simulink model "ctrl_systems_3"  (Simulink 10.2)
settings: Solver=ode45  StartTime=0.0  StopTime=365  MaxStep=0.01  RelTol=1e-3  EnableMultiTasking=on
values from neighbouring files (symbols this model uses):
  A = 10    [setup_Prac5.m]
  alpha = 0.1    [setup_Prac5.m]
  b1 = csvread('./DAE_ANN/ANN/Biases/30_04_21/lstm_ann_pi_standard_fix_noSo4_rnn_1__100_16_b_3.csv')    [init_PI_ann.m]    (also in init_PI_ann_hier.m = csvread('./DAE_ANN/ANN/Biases/12_05_21/lstm_ann_pi_standard_; init_PI_ann_hier_v2.m = csvread('./DAE_ANN/ANN/Biases/12_05_21/lstm_ann_pi_standard_; init_PI_ann_lab.m = csvread('./DAE_ANN/ANN/Biases/12_05_21/lstm_ann_pi_standard_)
  b2 = csvread('./DAE_ANN/ANN/Biases/30_04_21/lstm_ann_pi_standard_fix_noSo4_rnn_1__100_16_b_3.csv')    [init_PI_ann.m]    (also in init_PI_ann_hier.m = csvread('./DAE_ANN/ANN/Biases/12_05_21/lstm_ann_pi_standard_; init_PI_ann_hier_v2.m = csvread('./DAE_ANN/ANN/Biases/12_05_21/lstm_ann_pi_standard_; init_PI_ann_lab.m = csvread('./DAE_ANN/ANN/Biases/12_05_21/lstm_ann_pi_standard_)
  b_last = csvread('./DAE_ANN/ANN/Biases/12_05_21/lstm_ann_pi_standard_fix_noSo4_last__100_1_b_2.csv')'    [init_PI_ann_hier.m]    (also in init_PI_ann_hier_v2.m; init_PI_ann_lab.m)
  b_out = csvread('./DAE_ANN/ANN/Biases/30_04_21/lstm_ann_pi_standard_fix_noSo4_final__100_16_b_3.csv')    [init_PI_ann.m]    (also in init_PI_ann_hier.m = csvread('./DAE_ANN/ANN/Biases/12_05_21/lstm_ann_pi_standard_; init_PI_ann_hier_v2.m = csvread('./DAE_ANN/ANN/Biases/12_05_21/lstm_ann_pi_standard_; init_PI_ann_lab.m = csvread('./DAE_ANN/ANN/Biases/12_05_21/lstm_ann_pi_standard_)
  beta_ctrl = 0.3331    [setup_Prac5.m]
  k = k+1    (= 2)    [perf_risk.m]    (also in setup_Prac5.m = As*sqrt(2*g))
  K = 0.2294    [setup_Prac5.m]
  Kc_filter = 32.3841    [setup_Prac5.m]
  mean_scaler_dir = csvread('./DAE_ANN/ANN/Scalers/30_04_21_lstm_ann_pi_standard_fix_noSo4/mean_scaler_lstm_ann_pi_standard_fix_noSo4.csv')    [init_PI_ann.m]    (also in init_PI_ann_hier.m = csvread('./DAE_ANN/ANN/Scalers/12_05_21_lstm_ann_pi_standard; init_PI_ann_hier_v2.m = csvread('./DAE_ANN/ANN/Scalers/12_05_21_lstm_ann_pi_standard; setup_Prac5.m = [(Q/k)^2, 1.9756, 0.0000, 0]')
  mean_scaler_dir_out = csvread('./DAE_ANN/ANN/Scalers/30_04_21_lstm_ann_pi_standard_fix_noSo4/mean_scaler_lstm_ann_pi_standard_fix_noSo4_out.csv')    [init_PI_ann.m]    (also in init_PI_ann_hier.m = csvread('./DAE_ANN/ANN/Scalers/12_05_21_lstm_ann_pi_standard; init_PI_ann_hier_v2.m = csvread('./DAE_ANN/ANN/Scalers/12_05_21_lstm_ann_pi_standard; setup_Prac5.m = 0)
  n_layers = 1    [init_PI_ann.m]    (also in init_PI_ann_hier.m; init_PI_ann_hier_v2.m; init_PI_ann_lab.m)
  n_sw = 16    [init_PI_ann.m]    (also in init_PI_ann_hier.m = 1; init_PI_ann_hier_v2.m = 1; init_PI_ann_lab.m = 1)
  Q = 2    [setup_Prac5.m]
  So_mean = 2    [run_bsm1_PIANN_variable.m]    (also in setup_Prac5.m = 0.2)
  std_scaler_dir = csvread('./DAE_ANN/ANN/Scalers/30_04_21_lstm_ann_pi_standard_fix_noSo4/std_scaler_lstm_ann_pi_standard_fix_noSo4.csv')    [init_PI_ann.m]    (also in init_PI_ann_hier.m = csvread('./DAE_ANN/ANN/Scalers/12_05_21_lstm_ann_pi_standard; init_PI_ann_hier_v2.m = csvread('./DAE_ANN/ANN/Scalers/12_05_21_lstm_ann_pi_standard; setup_Prac5.m = [1, 0.7579, 0.05, 1]')
  std_scaler_dir_out = csvread('./DAE_ANN/ANN/Scalers/30_04_21_lstm_ann_pi_standard_fix_noSo4/std_scaler_lstm_ann_pi_standard_fix_noSo4_out.csv')    [init_PI_ann.m]    (also in init_PI_ann_hier.m = csvread('./DAE_ANN/ANN/Scalers/12_05_21_lstm_ann_pi_standard; init_PI_ann_hier_v2.m = csvread('./DAE_ANN/ANN/Scalers/12_05_21_lstm_ann_pi_standard; setup_Prac5.m = 1)
  T = 6.5201    [setup_Prac5.m]
  t_init = 7e-3    (= 0.007)    [run_bsm1.m]    (also in run_bsm1_PIANN_variable.m = 0.05)
  t_simulink = 1/96    (= 0.0104166666667)    [run_bsm1.m]    (also in run_bsm1_PIANN.m = -1; run_bsm1_PIANN_variable.m = 0; setup_Prac5.m = 0)
  Td_filter = 0.2776    [setup_Prac5.m]
  Ti_filter = 1.0264    [setup_Prac5.m]
  u1 = csvread('./DAE_ANN/ANN/Weights/30_04_21/lstm_ann_pi_standard_fix_noSo4_rnn_1__100_16_U_3.csv')    [init_PI_ann.m]    (also in init_PI_ann_hier.m = csvread('./DAE_ANN/ANN/Weights/12_05_21/lstm_ann_pi_standard; init_PI_ann_hier_v2.m = csvread('./DAE_ANN/ANN/Weights/12_05_21/lstm_ann_pi_standard)
  u2 = csvread('./DAE_ANN/ANN/Weights/30_04_21/lstm_ann_pi_standard_fix_noSo4_rnn_1__100_16_U_3.csv')    [init_PI_ann.m]    (also in init_PI_ann_hier.m = csvread('./DAE_ANN/ANN/Weights/12_05_21/lstm_ann_pi_standard; init_PI_ann_hier_v2.m = csvread('./DAE_ANN/ANN/Weights/12_05_21/lstm_ann_pi_standard)
  w1 = csvread('./DAE_ANN/ANN/Weights/30_04_21/lstm_ann_pi_standard_fix_noSo4_rnn_1__100_16_W_3.csv')    [init_PI_ann.m]    (also in init_PI_ann_hier.m = csvread('./DAE_ANN/ANN/Weights/12_05_21/lstm_ann_pi_standard; init_PI_ann_hier_v2.m = csvread('./DAE_ANN/ANN/Weights/12_05_21/lstm_ann_pi_standard; init_PI_ann_lab.m = csvread('./DAE_ANN/ANN/Weights/12_05_21/lstm_ann_pi_standard)
  w2 = csvread('./DAE_ANN/ANN/Weights/30_04_21/lstm_ann_pi_standard_fix_noSo4_rnn_1__100_16_W_3.csv')    [init_PI_ann.m]    (also in init_PI_ann_hier.m = csvread('./DAE_ANN/ANN/Weights/12_05_21/lstm_ann_pi_standard; init_PI_ann_hier_v2.m = csvread('./DAE_ANN/ANN/Weights/12_05_21/lstm_ann_pi_standard; init_PI_ann_lab.m = csvread('./DAE_ANN/ANN/Weights/12_05_21/lstm_ann_pi_standard)
  w_last = csvread('./DAE_ANN/ANN/Weights/12_05_21/lstm_ann_pi_standard_fix_noSo4_last__100_1_W_2.csv')    [init_PI_ann_hier.m]    (also in init_PI_ann_hier_v2.m; init_PI_ann_lab.m)
  w_out = csvread('./DAE_ANN/ANN/Weights/30_04_21/lstm_ann_pi_standard_fix_noSo4_final__100_16_W_3.csv')    [init_PI_ann.m]    (also in init_PI_ann_hier.m = csvread('./DAE_ANN/ANN/Weights/12_05_21/lstm_ann_pi_standard; init_PI_ann_hier_v2.m = csvread('./DAE_ANN/ANN/Weights/12_05_21/lstm_ann_pi_standard; init_PI_ann_lab.m = csvread('./DAE_ANN/ANN/Weights/12_05_21/lstm_ann_pi_standard)
  x0_ini = [2*(Q/k)^2  (Q/k)^2]    [setup_Prac5.m]
undefined symbols (not defined in the file or in its folder): Kc_zn, magnitude, Td_zn, Ti_zn
settings Model: Creator=carles  LastModifiedBy=win04
settings DataIOCC: OutputTimes=1
settings OptimizationCC: ExpressionDepthLimit=2147483647
settings DebuggingCC: SolverPrmCheckMsg=warning  StateNameClashWarn=warning
settings ConfigComp: CovSFcnEnable=off

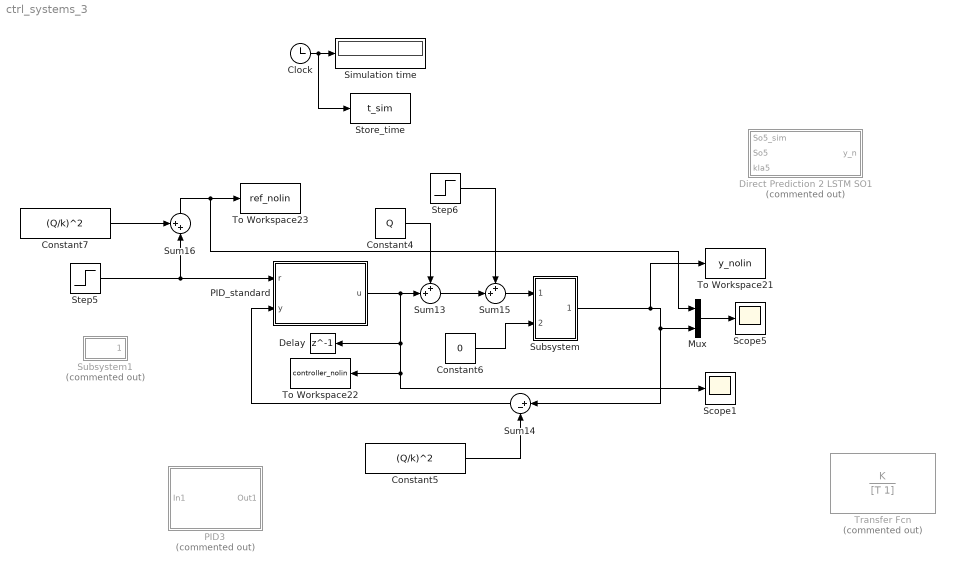
== system ctrl_systems_3 ==
  Clock : Clock
  Constant4 : Constant  Value=Q
  Constant5 : Constant  Value=(Q/k)^2
  Constant6 : Constant  Value=0
  Constant7 : Constant  Value=(Q/k)^2
  Delay : Delay  DelayLength=1  InitialCondition=0  SampleTime=0.0001
  Direct Prediction 2 LSTM SO1 : Subsystem  Commented=on
  Mux : Mux  Inputs=2
  PID3 : Subsystem  Commented=on
  PID_standard : Subsystem
  Scope1 : Scope
  Scope5 : Scope
  Simulation time : Display
  Step5 : Step  Time=5  After=0.2  SampleTime=0
  Step6 : Step  Time=30  After=0  SampleTime=0
  Store_time : ToWorkspace  VariableName=t_sim
  Subsystem : Subsystem
  Subsystem1 : Subsystem  Commented=on
  Sum13 : Sum  Inputs=++|
  Sum14 : Sum  Inputs=|+-
  Sum15 : Sum  Inputs=++|
  Sum16 : Sum  Inputs=++|
  To Workspace21 : ToWorkspace  VariableName=y_nolin  SampleTime=-1
  To Workspace22 : ToWorkspace  VariableName=controller_nolin  SampleTime=-1
  To Workspace23 : ToWorkspace  VariableName=ref_nolin  SampleTime=-1
  Transfer Fcn : TransferFcn  Commented=on  Numerator=K  Denominator=[T 1]
  wires:
  Subsystem/1(Out2) -> Sum14/1, Mux/2, To Workspace21/1
  Constant4/1 -> Sum13/1
  Constant5/1 -> Sum14/2
  PID_standard/1(u) -> Scope1/1, To Workspace22/1, Delay/1, Sum13/2
  Sum15/1 -> Subsystem/1(In1)
  Sum13/1 -> Sum15/2
  Step5/1 -> PID_standard/1(r), Sum16/2
  Step6/1 -> Sum15/1
  Sum16/1 -> Mux/1, To Workspace23/1
  Constant7/1 -> Sum16/1
  Clock/1 -> Store_time/1, Simulation time/1
  Sum14/1 -> PID_standard/2(y)
  Mux/1 -> Scope5/1
  Constant6/1 -> Subsystem/2(In2)

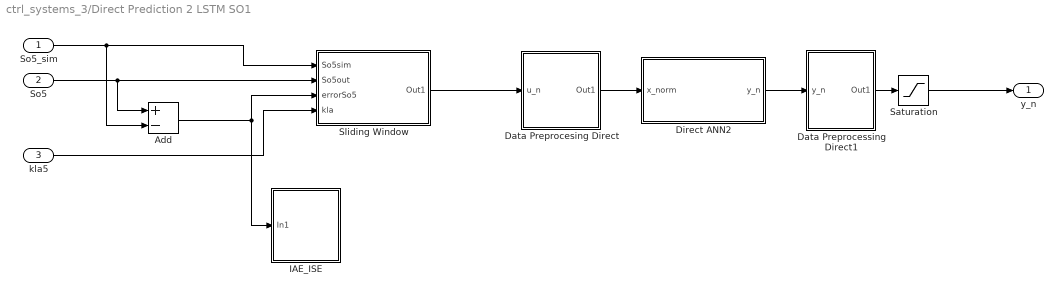
== system ctrl_systems_3/Direct Prediction 2 LSTM SO1 ==
  So5_sim : Inport
  So5 : Inport  Port=2
  kla5 : Inport  Port=3
  Add : Sum  Inputs=+-
  Data Preprocesing Direct : Subsystem
  Data Preprocessing Direct1 : Subsystem
  Direct ANN2 : Subsystem
  IAE_ISE : Subsystem
  Saturation : Saturate  UpperLimit=360  LowerLimit=-Q
  Sliding Window : Subsystem
  y_n : Outport  VectorParamsAs1DForOutWhenUnconnected=off
  wires:
  kla5/1 -> Sliding Window/4(kla)
  Add/1 -> Sliding Window/3(errorSo5), IAE_ISE/1(In1)
  So5/1 -> Sliding Window/2(So5out), Add/1
  So5_sim/1 -> Sliding Window/1(So5sim), Add/2
  Saturation/1 -> y_n/1
  Sliding Window/1(Out1) -> Data Preprocesing Direct/1(u_n)
  Data Preprocessing Direct1/1(Out1) -> Saturation/1
  Direct ANN2/1(y_n) -> Data Preprocessing Direct1/1(y_n)
  Data Preprocesing Direct/1(Out1) -> Direct ANN2/1(x_norm)

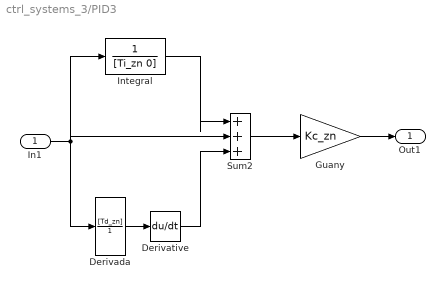
== system ctrl_systems_3/PID3 ==
  In1 : Inport
  Derivada : TransferFcn  Numerator=[Td_zn]  Denominator=[1]
  Derivative : Derivative
  Guany : Gain  Gain=Kc_zn
  Integral : TransferFcn  Denominator=[Ti_zn 0]
  Sum2 : Sum  Inputs=|+++
  Out1 : Outport
  wires:
  Derivative/1 -> Sum2/3
  Derivada/1 -> Derivative/1
  In1/1 -> Integral/1, Derivada/1, Sum2/2
  Integral/1 -> Sum2/1
  Sum2/1 -> Guany/1
  Guany/1 -> Out1/1

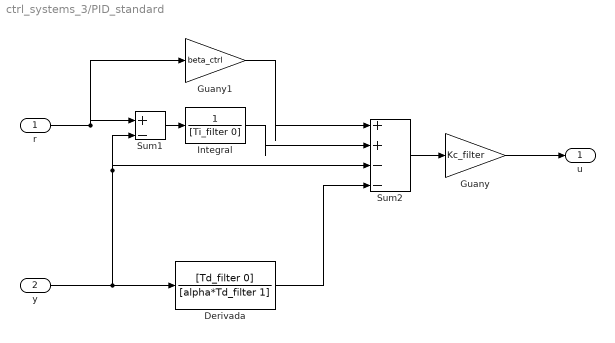
== system ctrl_systems_3/PID_standard ==
  r : Inport
  y : Inport  Port=2
  Derivada : TransferFcn  Numerator=[Td_filter 0]  Denominator=[alpha*Td_filter 1]
  Guany : Gain  Gain=Kc_filter
  Guany1 : Gain  Gain=beta_ctrl
  Integral : TransferFcn  Denominator=[Ti_filter 0]
  Sum1 : Sum  Inputs=|+-
  Sum2 : Sum  Inputs=|++--
  u : Outport
  wires:
  Guany/1 -> u/1
  Sum2/1 -> Guany/1
  r/1 -> Sum1/1, Guany1/1
  Guany1/1 -> Sum2/1
  Integral/1 -> Sum2/2
  y/1 -> Derivada/1, Sum2/3, Sum1/2
  Derivada/1 -> Sum2/4
  Sum1/1 -> Integral/1

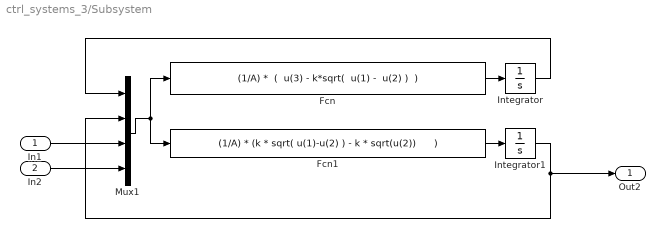
== system ctrl_systems_3/Subsystem ==
  In1 : Inport
  In2 : Inport  Port=2
  Fcn : Fcn  Expr="(1/A) *  (  u(3) - k*sqrt(  u(1) -  u(2) )  )"
  Fcn1 : Fcn  Expr="(1/A) * (k * sqrt( u(1)-u(2) ) - k * sqrt(u(2))      )"
  Integrator : Integrator  InitialCondition=x0_ini(1)
  Integrator1 : Integrator  InitialCondition=x0_ini(2)
  Mux1 : Mux
  Out2 : Outport
  wires:
  In1/1 -> Mux1/3
  In2/1 -> Mux1/4
  Integrator1/1 -> Out2/1, Mux1/2
  Integrator/1 -> Mux1/1
  Mux1/1 -> Fcn/1, Fcn1/1
  Fcn1/1 -> Integrator1/1
  Fcn/1 -> Integrator/1

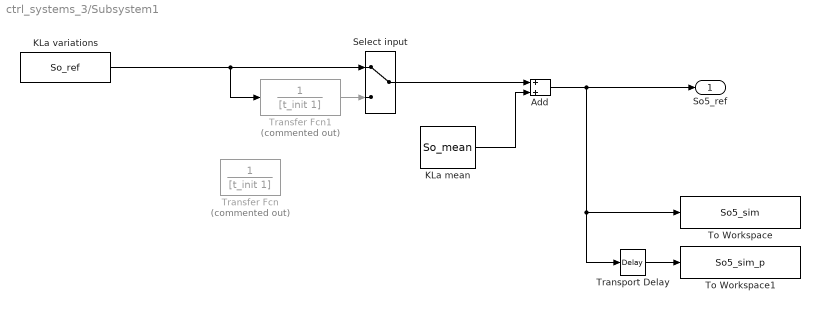
== system ctrl_systems_3/Subsystem1 ==
  Add : Sum
  KLa mean : Constant  Value=So_mean
  KLa variations : FromWorkspace  VariableName=So_ref  SampleTime=-1  ZeroCross=off  OutputAfterFinalValue=Holding final value
  Select input : ManualSwitch
  To Workspace : ToWorkspace  VariableName=So5_sim  SampleTime=t_simulink
  To Workspace1 : ToWorkspace  VariableName=So5_sim_p  SampleTime=t_simulink
  Transfer Fcn : TransferFcn  Commented=on  Denominator=[t_init 1]
  Transfer Fcn1 : TransferFcn  Commented=on  Denominator=[t_init 1]
  Transport Delay : TransportDelay  DelayTime=10/(60*24)
  So5_ref : Outport  VectorParamsAs1DForOutWhenUnconnected=off
  wires:
  Transport Delay/1 -> To Workspace1/1
  KLa variations/1 -> Select input/1, Transfer Fcn1/1
  Transfer Fcn1/1 -> Select input/2
  Select input/1 -> Add/1
  Add/1 -> To Workspace/1, Transport Delay/1, So5_ref/1
  KLa mean/1 -> Add/2

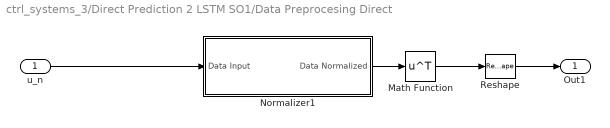
== system ctrl_systems_3/Direct Prediction 2 LSTM SO1/Data Preprocesing Direct ==
  u_n : Inport
  Math Function : Math  Operator=transpose  SignedPower=on  SaturateOnIntegerOverflow=on
  Normalizer1 : Subsystem
  Reshape : Reshape  OutputDimensionality=Row vector (2-D)
  Out1 : Outport  VectorParamsAs1DForOutWhenUnconnected=off
  wires:
  u_n/1 -> Normalizer1/1(Data Input)
  Math Function/1 -> Reshape/1
  Normalizer1/1(Data Normalized) -> Math Function/1
  Reshape/1 -> Out1/1

== system ctrl_systems_3/Direct Prediction 2 LSTM SO1/Data Preprocessing Direct1 ==
  y_n : Inport
  Denormalization Values : MATLAB Function  TreatAsAtomicUnit=on
  Out1 : Outport  VectorParamsAs1DForOutWhenUnconnected=off
  wires:
  Denormalization Values/1(data_dir) -> Out1/1
  y_n/1 -> Denormalization Values/1(data_input)

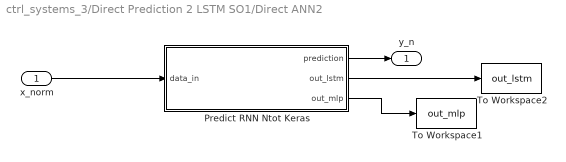
== system ctrl_systems_3/Direct Prediction 2 LSTM SO1/Direct ANN2 ==
  x_norm : Inport
  Predict RNN Ntot Keras : MATLAB Function  TreatAsAtomicUnit=on
  To Workspace1 : ToWorkspace  VariableName=out_mlp  SampleTime=-1
      settings: Save2DSignal=2-D array (concatenate along first dimension)
  To Workspace2 : ToWorkspace  VariableName=out_lstm  SampleTime=-1
      settings: Save2DSignal=2-D array (concatenate along first dimension)
  y_n : Outport  VectorParamsAs1DForOutWhenUnconnected=off
  wires:
  x_norm/1 -> Predict RNN Ntot Keras/1(data_in)
  Predict RNN Ntot Keras/1(prediction) -> y_n/1
  Predict RNN Ntot Keras/2(out_lstm) -> To Workspace2/1
  Predict RNN Ntot Keras/3(out_mlp) -> To Workspace1/1

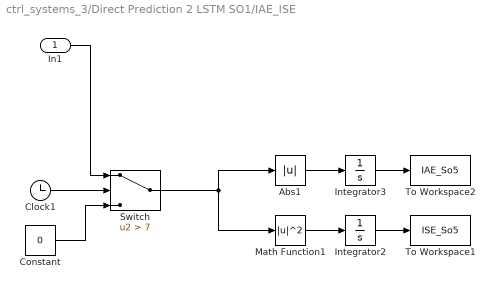
== system ctrl_systems_3/Direct Prediction 2 LSTM SO1/IAE_ISE ==
  In1 : Inport
  Abs1 : Abs
  Clock1 : Clock
  Constant : Constant  Value=0
  Integrator2 : Integrator
  Integrator3 : Integrator
  Math Function1 : Math  Operator=magnitude^2  SignedPower=on  SaturateOnIntegerOverflow=on
  Switch : Switch  Criteria=u2 > Threshold  Threshold=7
  To Workspace1 : ToWorkspace  VariableName=ISE_So5  SampleTime=-1
  To Workspace2 : ToWorkspace  VariableName=IAE_So5  SampleTime=-1
  wires:
  Clock1/1 -> Switch/2
  Abs1/1 -> Integrator3/1
  In1/1 -> Switch/1
  Constant/1 -> Switch/3
  Integrator3/1 -> To Workspace2/1
  Integrator2/1 -> To Workspace1/1
  Switch/1 -> Math Function1/1, Abs1/1
  Math Function1/1 -> Integrator2/1

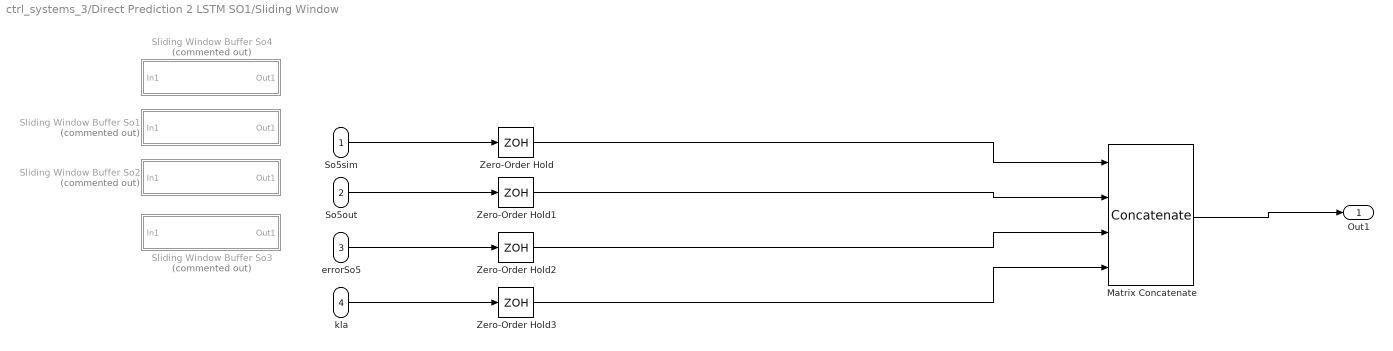
== system ctrl_systems_3/Direct Prediction 2 LSTM SO1/Sliding Window ==
  So5sim : Inport
  So5out : Inport  Port=2
  errorSo5 : Inport  Port=3
  kla : Inport  Port=4
  Matrix Concatenate : Concatenate  NumInputs=4  Mode=Multidimensional array  ConcatenateDimension=2
  Sliding Window Buffer So1 : Subsystem  Commented=on
  Sliding Window Buffer So2 : Subsystem  Commented=on
  Sliding Window Buffer So3 : Subsystem  Commented=on
  Sliding Window Buffer So4 : Subsystem  Commented=on
  Zero-Order Hold{,1..3} (4 alike) : ZeroOrderHold  SampleTime=-1
  Out1 : Outport
  wires:
  Zero-Order Hold3/1 -> Matrix Concatenate/4
  Zero-Order Hold2/1 -> Matrix Concatenate/3
  Zero-Order Hold1/1 -> Matrix Concatenate/2
  Zero-Order Hold/1 -> Matrix Concatenate/1
  kla/1 -> Zero-Order Hold3/1
  errorSo5/1 -> Zero-Order Hold2/1
  So5out/1 -> Zero-Order Hold1/1
  So5sim/1 -> Zero-Order Hold/1
  Matrix Concatenate/1 -> Out1/1

== system ctrl_systems_3/Direct Prediction 2 LSTM SO1/Data Preprocesing Direct/Normalizer1 ==
  Data Input : Inport
  Normalization Values : MATLAB Function  TreatAsAtomicUnit=on
  Data Normalized : Outport  VectorParamsAs1DForOutWhenUnconnected=off
  wires:
  Data Input/1 -> Normalization Values/1(data_input)
  Normalization Values/1(data_norm) -> Data Normalized/1

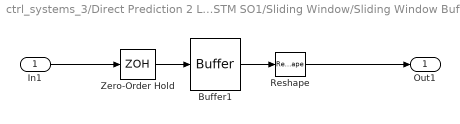
== system ctrl_systems_3/Direct Prediction 2 LSTM SO1/Sliding Window/Sliding Window Buffer So1 ==
  In1 : Inport
  Buffer1 : Buffer  N=16  V=15
  Reshape : Reshape
  Zero-Order Hold : ZeroOrderHold  SampleTime=1/96
  Out1 : Outport
  wires:
  Zero-Order Hold/1 -> Buffer1/1
  In1/1 -> Zero-Order Hold/1
  Reshape/1 -> Out1/1
  Buffer1/1 -> Reshape/1

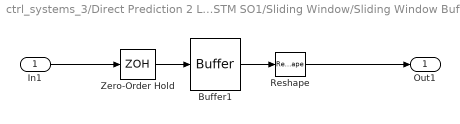
== system ctrl_systems_3/Direct Prediction 2 LSTM SO1/Sliding Window/Sliding Window Buffer So2 ==
  In1 : Inport
  Buffer1 : Buffer  N=16  V=15
  Reshape : Reshape
  Zero-Order Hold : ZeroOrderHold  SampleTime=1/96
  Out1 : Outport
  wires:
  Zero-Order Hold/1 -> Buffer1/1
  In1/1 -> Zero-Order Hold/1
  Reshape/1 -> Out1/1
  Buffer1/1 -> Reshape/1

== system ctrl_systems_3/Direct Prediction 2 LSTM SO1/Sliding Window/Sliding Window Buffer So3 ==
  In1 : Inport
  Buffer1 : Buffer  N=16  V=15
  Reshape : Reshape
  Zero-Order Hold : ZeroOrderHold  SampleTime=-1
  Out1 : Outport
  wires:
  Zero-Order Hold/1 -> Buffer1/1
  In1/1 -> Zero-Order Hold/1
  Reshape/1 -> Out1/1
  Buffer1/1 -> Reshape/1

== system ctrl_systems_3/Direct Prediction 2 LSTM SO1/Sliding Window/Sliding Window Buffer So4 ==
  In1 : Inport
  Buffer1 : Buffer  N=16  V=15
  Reshape : Reshape
  Zero-Order Hold : ZeroOrderHold  SampleTime=1/96
  Out1 : Outport
  wires:
  Zero-Order Hold/1 -> Buffer1/1
  In1/1 -> Zero-Order Hold/1
  Reshape/1 -> Out1/1
  Buffer1/1 -> Reshape/1

== matlab function Direct Prediction 2 LSTM SO1/Data Preprocesing Direct/Normalizer1/Normalization Values ==
  data: mean_scaler_dir parameter double; data_norm output double; std_scaler_dir parameter double; data_input input double
function data_norm = scaler(mean_scaler_dir, std_scaler_dir, data_input)
%#codegen

mean_output_2 = mean_scaler_dir';
std_output_2 = std_scaler_dir';

data_norm = (data_input - mean_output_2)./std_output_2;

== matlab function Direct Prediction 2 LSTM SO1/Direct ANN2/Predict RNN Ntot Keras ==
  data: data_in input double; prediction output double; w1 parameter double; u1 parameter double; w2 parameter double; u2 parameter double; b1 parameter double; b2 parameter double; w_out parameter double; b_out parameter double; n_layers parameter double; n_sw parameter double; w_last parameter double; b_last parameter double; out_lstm output double; out_mlp output double
function [prediction, out_lstm, out_mlp]= predict_rnn(data_in, w1, u1, w2, u2, b1, b2, w_out, b_out, n_layers, n_sw, w_last, b_last)
%#codegen
    
    prediction = 0;
    
    dim_w1 = size(w1);
    dim_w2 = size(w2);
    n_input = dim_w1(1);
    n_steps = n_sw;
    n_hidden = dim_w1(2)/4;
    n_hidden_2 = 50;
    
    %% Layer 1

    w_i_1 = w1(:,1:n_hidden);
    w_f_1 = w1(:,n_hidden*1+1:n_hidden*2);
    w_C_1 = w1(:,n_hidden*2+1:n_hidden*3);
    w_o_1 = w1(:,n_hidden*3+1:end);

    u_i_1 = u1(:,1:n_hidden);
    u_f_1 = u1(:,n_hidden*1+1:n_hidden*2);
    u_C_1 = u1(:,n_hidden*2+1:n_hidden*3);
    u_o_1 = u1(:,n_hidden*3+1:end);
   
    b_i_1 = b1(1:n_hidden)';
    b_f_1 = b1(n_hidden*1+1:n_hidden*2)';
    b_C_1 = b1(n_hidden*2+1:n_hidden*3)';
    b_o_1 = b1(n_hidden*3+1:n_hidden*4)';

%% Layer 2

    w_i_2 = w2(:,1:n_hidden_2);
    w_f_2 = w2(:,n_hidden_2*1+1:n_hidden_2*2);
    w_C_2 = w2(:,n_hidden_2*2+1:n_hidden_2*3);
    w_o_2 = w2(:,n_hidden_2*3+1:end);

    u_i_2 = u2(:,1:n_hidden_2);
    u_f_2 = u2(:,n_hidden_2*1+1:n_hidden_2*2);
    u_C_2 = u2(:,n_hidden_2*2+1:n_hidden_2*3);
    u_o_2 = u2(:,n_hidden_2*3+1:end);
    
    b_i_2 = b2(1:n_hidden_2)';
    b_f_2 = b2(n_hidden_2+1:n_hidden_2*2)';
    b_C_2 = b2(n_hidden_2*2+1:n_hidden_2*3)';
    b_o_2 = b2(n_hidden_2*3+1:n_hidden_2*4)';

%% Split data in four parts
                 
    j = 1;
        
    h_t1 = zeros(1, n_hidden);
    C_t1 = zeros(1, n_hidden);

    h_t2 = zeros(1, n_hidden_2);
    C_t2 = zeros(1, n_hidden_2);
    
    prediction_aux_v2 = zeros(1, n_hidden_2/2);

    out_lstm = zeros(1, n_hidden_2);

    out_mlp = prediction_aux_v2;
    
    prediction_aux = 0;
    

    while j<=n_steps
        
        x_t = data_in(1+n_input*(j-1):n_input*j);
            
        f_t_1_nosig = ((x_t*w_f_1)+(h_t1*u_f_1)+(b_f_1));
        f_t_1 = 1./(1 + exp(-1.*(f_t_1_nosig)));
        i_t_1_nosig = ((x_t*w_i_1)+(h_t1*u_i_1)+b_i_1);
        i_t_1 = 1./(1 + exp(-1.*(i_t_1_nosig)));
        C_t1_new = tanh((x_t*w_C_1)+(h_t1*u_C_1)+b_C_1);
        C_t1 = (f_t_1).*C_t1 + i_t_1.*C_t1_new;
            
        o_t_1_nosig = ((x_t*w_o_1)+(h_t1*u_o_1)+b_o_1);
        o_t_1 = 1./(1 + exp(-1.*(o_t_1_nosig)));
        h_t1 = o_t_1.*tanh(C_t1);
        
        f_t_2_nosig = ((h_t1*w_f_2)+(h_t2*u_f_2)+(b_f_2+1));
        f_t_2 = 1./(1 + exp(-1.*(f_t_2_nosig)));
        i_t_2_nosig = ((h_t1*w_i_2)+(h_t2*u_i_2)+b_i_2);
        i_t_2 = 1./(1 + exp(-1.*(i_t_2_nosig)));
        C_t2_new = tanh((h_t1*w_C_2)+(h_t2*u_C_2)+b_C_2);
        C_t2 = f_t_2.*C_t2 + i_t_2.*C_t2_new;

        o_t_2_nosig = ((h_t1*w_o_2)+(h_t2*u_o_2)+b_o_2);
        o_t_2 = 1./(1 + exp(-1.*(o_t_2_nosig)));
        h_t2 = o_t_2.*tanh(C_t2);    

        prediction_aux_2 = h_t2*w_last + b_last;
        
        prediction_aux_2(prediction_aux_2<0) = 0;
        
        prediction_aux = prediction_aux_2*w_out + b_out;

                        
        j = j+1;
    end
    
    out_mlp = prediction_aux_2;
    out_lstm = h_t2;
    prediction = prediction_aux;
end

== matlab function Direct Prediction 2 LSTM SO1/Data Preprocessing Direct1/Denormalization Values ==
  data: mean_scaler_dir_out parameter double; data_dir output double; std_scaler_dir_out parameter double; data_input input double
function data_dir = descaler(mean_scaler_dir_out, std_scaler_dir_out, data_input)
%#codegen

mean_output_2 = mean_scaler_dir_out;
std_output_2 = std_scaler_dir_out;

data_dir = std_output_2.*data_input + mean_output_2;
